simulink model "Lab2_P2Q1f"  (R2019a)
settings: Solver=FixedStepDiscrete  StartTime=0.0  StopTime=10.0  FixedStep=0.01  RelTol=1e-3
libraries: simulink_extras x1
settings Model: Creator=keeshigan  LastModifiedBy=pmangat5

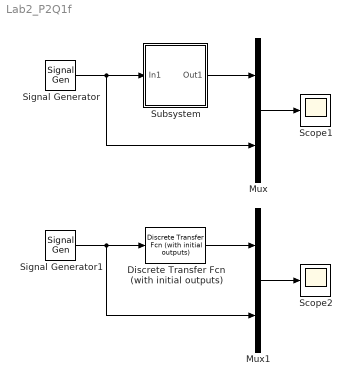
== system Lab2_P2Q1f ==
  Discrete Transfer Fcn (with initial outputs) : simulink_extras/Additional Discrete/Discrete Transfer Fcn (with initial outputs)  N=[0.01]  D="[1  -1]"  U0=[1]  Y0=0  TS=0.01
      settings: SourceProductName=Simulink  SourceProductBaseCode=SL
  Mux : Mux  Inputs=2
  Mux1 : Mux  Inputs=2
  Scope1 : Scope
  Scope2 : Scope
  Signal Generator : SignalGenerator
  Signal Generator1 : SignalGenerator
  Subsystem : Subsystem
  wires:
  Subsystem/1(Out1) -> Mux/1
  Mux/1 -> Scope1/1
  Signal Generator/1 -> Mux/2, Subsystem/1(In1)
  Mux1/1 -> Scope2/1
  Discrete Transfer Fcn (with initial outputs)/1 -> Mux1/1
  Signal Generator1/1 -> Discrete Transfer Fcn (with initial outputs)/1, Mux1/2

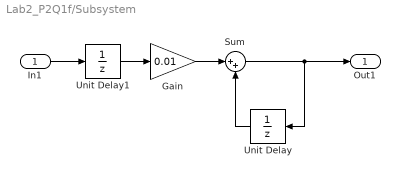
== system Lab2_P2Q1f/Subsystem ==
  In1 : Inport
  Gain : Gain  Gain=0.01
  Sum : Sum  Inputs=|++
  Unit Delay : UnitDelay  SampleTime=-1  HasFrameUpgradeWarning=on
  Unit Delay1 : UnitDelay  SampleTime=-1  HasFrameUpgradeWarning=on
  Out1 : Outport  VectorParamsAs1DForOutWhenUnconnected=on
  wires:
  Unit Delay1/1 -> Gain/1
  Unit Delay/1 -> Sum/2
  In1/1 -> Unit Delay1/1
  Gain/1 -> Sum/1
  Sum/1 -> Out1/1, Unit Delay/1
